simulink model "ICE_Model"  (R2020a)
settings: Solver=VariableStepAuto  StartTime=0.0  StopTime=6948  RelTol=1e-3
libraries: qss_tb_library x6
settings Model: Creator=patri  LastModifiedBy=Rahul Pai

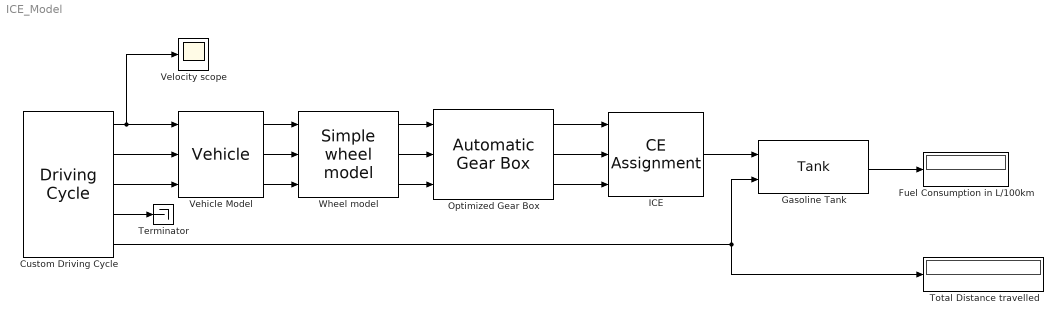
== system ICE_Model ==
  Custom Driving Cycle : qss_tb_library/Driving Cycle/Driving Cycle  Tag=cycle  cyclename1=Assignment_2_cycle  stepsize=1  autostop=on
  Fuel Consumption in L/100km : Display
  Gasoline Tank : qss_tb_library/Energy Source/Tank  Tag=tank  fuel=Gasoline  flag_cold_start=on
  ICE : qss_tb_library/Energy Converter/CE Assignment  Tag=combustion engine  engine_type=Gasoline  P_ice=max_CE_power  ENABLE_FUEL_CUTOFF=on
  Optimized Gear Box : qss_tb_library/Gear System/Automatic Gear Box  Tag=transmission  nog=Gears  i=gear_ratio  i_diff=diff_gear  gearon=gear_up  gearoff=gear_down  d=V_wheel_dia  e_GT=gear_eff  P_GT0=gear_idling_loss  w_wheel_min=1
  Terminator : Terminator
  Total Distance travelled : Display
  Vehicle Model : qss_tb_library/Vehicle/Vehicle  Tag=vehicle  m_f=V_Mass  A_f=V_area  cw=V_d  mu=V_RRC  k_inertia=V_Rotating
  Velocity scope : Scope
  Wheel model : qss_tb_library/Vehicle/Simple wheel model  Tag=simple transmission  d_wheel=V_wheel_dia
  wires:
  Custom Driving Cycle/1 -> Velocity scope/1, Vehicle Model/1
  Custom Driving Cycle/2 -> Vehicle Model/2
  Custom Driving Cycle/3 -> Vehicle Model/3
  Vehicle Model/1 -> Wheel model/1
  Vehicle Model/2 -> Wheel model/2
  Vehicle Model/3 -> Wheel model/3
  Wheel model/2 -> Optimized Gear Box/2
  Wheel model/3 -> Optimized Gear Box/3
  Wheel model/1 -> Optimized Gear Box/1
  Optimized Gear Box/1 -> ICE/1
  Optimized Gear Box/2 -> ICE/2
  Optimized Gear Box/3 -> ICE/3
  ICE/1 -> Gasoline Tank/1
  Custom Driving Cycle/4 -> Terminator/1
  Custom Driving Cycle/5 -> Total Distance travelled/1, Gasoline Tank/2
  Gasoline Tank/1 -> Fuel Consumption in L/100km/1
